simulink model "LoadFlow116BusNetwork_original"  (R2024a)
settings: Solver=FixedStepDiscrete  StartTime=0.0  StopTime=4.5  FixedStep=75e-6  RelTol=1e-3  EnableMultiTasking=on
undefined symbols (not defined in the file or in its folder): D1, D11, Delta
libraries: spsSeriesRLCBranchLib x164, spsLoadFlowBusLib x116, spsDistributedParametersLineLib x79, spsThreePhaseSeriesRLCLoadLib x60, spsThreePhaseTransformerTwoWindingsLib x52, spsThreePhaseParallelRLCLoadLib x44, spsThreePhaseVIMeasurementLib x44, spsSynchronousMachinepuStandardLib x28, spsExcitationSystemLib x28, spsHydraulicTurbineandGovernorLib x28, spsGenericPowerSystemStabilizerLib x28, spsMultiBandPowerSystemStabilizerLib x28
(part 3 of 15)

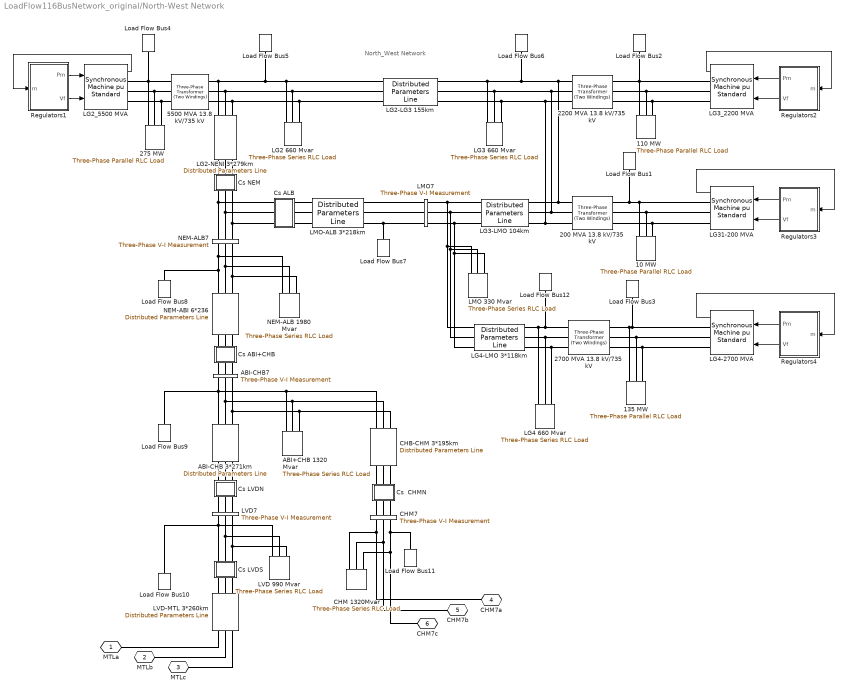
== system LoadFlow116BusNetwork_original/North-West Network ==
  note: North_West Network
  10 MW : spsThreePhaseParallelRLCLoadLib/Three-Phase Parallel RLC Load  LConnTagsString=A|B|C  Configuration=Y (grounded)  NominalVoltage=(13800)*1  Vabc=[1e3 1e3 1e3]  Vabcp=[1e3 1e3 1e3]  NominalFrequency=60  UnbalancedPower=off  ActivePower=10000000  InductivePower=0  CapacitivePower=0  Pabc=[10e3 9e3 11e3]  QLabc=[100 90 110]  QCabc=[100 90 110]  Pabcp=[10e3 9e3 11e3]  QLabcp=[100 90 110]  QCabcp=[100 90 110]  Measurements=None  LoadType=constant PQ
  110 MW : spsThreePhaseParallelRLCLoadLib/Three-Phase Parallel RLC Load  LConnTagsString=A|B|C  Configuration=Y (grounded)  NominalVoltage=(13800)*1  Vabc=[1e3 1e3 1e3]  Vabcp=[1e3 1e3 1e3]  NominalFrequency=60  UnbalancedPower=off  ActivePower=110000000  InductivePower=0  CapacitivePower=0  Pabc=[10e3 9e3 11e3]  QLabc=[100 90 110]  QCabc=[100 90 110]  Pabcp=[10e3 9e3 11e3]  QLabcp=[100 90 110]  QCabcp=[100 90 110]  Measurements=None  LoadType=constant PQ
  135 MW : spsThreePhaseParallelRLCLoadLib/Three-Phase Parallel RLC Load  LConnTagsString=A|B|C  Configuration=Y (grounded)  NominalVoltage=(13800)*1  Vabc=[1e3 1e3 1e3]  Vabcp=[1e3 1e3 1e3]  NominalFrequency=60  UnbalancedPower=off  ActivePower=135000000  InductivePower=0  CapacitivePower=0  Pabc=[10e3 9e3 11e3]  QLabc=[100 90 110]  QCabc=[100 90 110]  Pabcp=[10e3 9e3 11e3]  QLabcp=[100 90 110]  QCabcp=[100 90 110]  Measurements=None  LoadType=constant PQ
  200 MVA 13.8 kV/735 kV : spsThreePhaseTransformerTwoWindingsLib/Three-Phase Transformer (Two Windings)  Winding1Connection=Delta (D1)  Winding2Connection=Yg  CoreType=Three single-phase transformers  SetSaturation=off  Hysteresis=off  DataFile='basic_model'  SetInitialFlux=off  Measurements=None  UNITS=pu  NominalPower=[ 200e6 60 ]  Winding1="[ 13.8e3 0.002  0.0]"  Winding2=[ 735e3 0.002 0.12]  Rm=500  Lm=500  L0=0.5  Saturation="[ 0,0  ;  0.005,1.2  ;  1.0,1.4 ]"  InitialFluxes=[ 0.8 , -0.8 , 0.7 ]  BreakLoop=off  DiscreteSolver=Trapezoidal iterative  DataType=off  TransfoNumber=0
  2200 MVA 13.8 kV/735 kV : spsThreePhaseTransformerTwoWindingsLib/Three-Phase Transformer (Two Windings)  Winding1Connection=Delta (D1)  Winding2Connection=Yg  CoreType=Three single-phase transformers  SetSaturation=off  Hysteresis=off  DataFile='basic_model'  SetInitialFlux=off  Measurements=None  UNITS=pu  NominalPower=[ 2200e6 60 ]  Winding1="[ 13.8e3 0.002  0.0]"  Winding2=[ 735e3 0.002 0.12]  Rm=500  Lm=500  L0=0.5  Saturation="[ 0,0  ;  0.005,1.2  ;  1.0,1.4 ]"  InitialFluxes=[ 0.8 , -0.8 , 0.7 ]  BreakLoop=off  DiscreteSolver=Trapezoidal iterative  DataType=off  TransfoNumber=0
  2700 MVA 13.8 kV/735 kV : spsThreePhaseTransformerTwoWindingsLib/Three-Phase Transformer (Two Windings)  Winding1Connection=Delta (D1)  Winding2Connection=Yg  CoreType=Three single-phase transformers  SetSaturation=off  Hysteresis=off  DataFile='basic_model'  SetInitialFlux=off  Measurements=None  UNITS=pu  NominalPower=[ 2700e6 60 ]  Winding1="[ 13.8e3 0.002  0.0]"  Winding2=[ 735e3 0.002 0.12]  Rm=500  Lm=500  L0=0.5  Saturation="[ 0,0  ;  0.005,1.2  ;  1.0,1.4 ]"  InitialFluxes=[ 0.8 , -0.8 , 0.7 ]  BreakLoop=off  DiscreteSolver=Trapezoidal iterative  DataType=off  TransfoNumber=0
  275 MW : spsThreePhaseParallelRLCLoadLib/Three-Phase Parallel RLC Load  LConnTagsString=A|B|C  Configuration=Y (grounded)  NominalVoltage=(13800)*1  Vabc=[1e3 1e3 1e3]  Vabcp=[1e3 1e3 1e3]  NominalFrequency=60  UnbalancedPower=off  ActivePower=275000000  InductivePower=0  CapacitivePower=0  Pabc=[10e3 9e3 11e3]  QLabc=[100 90 110]  QCabc=[100 90 110]  Pabcp=[10e3 9e3 11e3]  QLabcp=[100 90 110]  QCabcp=[100 90 110]  Measurements=None  LoadType=constant PQ
  5500 MVA 13.8 kV/735 kV : spsThreePhaseTransformerTwoWindingsLib/Three-Phase Transformer (Two Windings)  Winding1Connection=Delta (D1)  Winding2Connection=Yg  CoreType=Three single-phase transformers  SetSaturation=off  Hysteresis=off  DataFile='basic_model'  SetInitialFlux=off  Measurements=None  UNITS=pu  NominalPower=[ 5500e6 60 ]  Winding1="[ 13.8e3 0.002  0.0]"  Winding2=[ 735e3 0.002 0.12]  Rm=500  Lm=500  L0=0.5  Saturation="[ 0,0  ;  0.005,1.2  ;  1.0,1.4 ]"  InitialFluxes=[ 0.8 , -0.8 , 0.7 ]  BreakLoop=off  DiscreteSolver=Trapezoidal iterative  DataType=off  TransfoNumber=0
  ABI+CHB 1320 Mvar : spsThreePhaseSeriesRLCLoadLib/Three-Phase Series RLC Load  LConnTagsString=A|B|C  Configuration=Y (grounded)  NominalVoltage=735e3  Vabc=[1e3 1e3 1e3]  Vabcp=[1e3 1e3 1e3]  NominalFrequency=60  UnbalancedPower=off  ActivePower=4400000  InductivePower=1320e6  CapacitivePower=0  Pabc=[10e3 9e3 11e3]  QLabc=[100 90 110]  QCabc=[100 90 110]  Pabcp=[10e3 9e3 11e3]  QLabcp=[100 90 110]  QCabcp=[100 90 110]  Measurements=None  LoadType=constant Z
  ABI-CHB 3*271km : spsDistributedParametersLineLib/Distributed Parameters Line  Phases=3  Length=271  Frequency=60  Resistance="[0.01273  0.3864]/3"  Inductance="[0.9337e-3  4.1264e-3]/3"  Capacitance=[12.74e-9 7.751e-9]*3  x1=[-0.001575 3.83249072532594e-08 -6095.79039966501 -646119.037388301;-0.0015 3.82765773827991e-08 12172.7797950193 -646033.103735147;-0.001425 3.81976498020301e-08 30431.6192557852 -645430.741103505;-0.00135 3.80881876044531e-08 48666.1321457375 -644312.431012847;-0.001275 3.79482782924739e-08 66861.7420742692 -642679.067423147;-0.0012 3.77780337074559e-08 85003.9037492058 -640531.956020269;-0.001125 3.75775899403154e-08 103078.114604089 -637872.813172216;-0.00105 3.7347107222733e-08 121069.926391305 -634703.764557095;-0.000975 3.70867697990666e-08 138964.956731796 -631027.343463879;-0.0009 3.67967857790695e-08 156748.900612111 -626846.488767341;-0.000825 3.64773869715303e-08 174407.541819615 -622164.542578755;-0.00075 3.61288286989688e-08 191926.764306713 -616985.247574268;-0.000675 3.5751389593535e-08 209292.563475003 -611312.744003061;-0.0006 3.53453713742747e-08 226491.057370334 -605151.566377697;-0.000525 3.49110986059401e-08 243508.497779833 -598506.6398493;-0.00045 3.44489184395376e-08 260331.281222011 -591383.276270467;-0.000375 3.39592003348207e-08 276945.959821183 -583787.16994905;-0.0003 3.34423357649494e-08 293339.252057489 -575724.393096219;-0.000225 3.28987379035524e-08 309498.053383942 -567201.390972425;-0.00015 3.23288412944429e-08 325409.446701998 -558224.976735161;-7.5e-05 3.17331015042505e-08 341060.712687292 -548802.325992623]  x2=[-0.001575 8.2065527540125e-08 -248614.692980884 -602078.188381389;-0.0015 8.19104771840523e-08 -231494.235349716 -608866.016701668;-0.001425 8.1689948845791e-08 -214188.724768791 -615167.126844157;-0.00135 8.14041188123205e-08 -196711.994998483 -620976.48179782;-0.001275 8.10532155717962e-08 -179078.016669168 -626289.437653192;-0.0012 8.06375196308996e-08 -161300.886113313 -631101.747314655;-0.001125 8.01573632906055e-08 -143394.814097085 -635409.563895494;-0.00105 7.96131303805457e-08 -125374.114460482 -639209.443793048;-0.000975 7.90052559521814e-08 -107253.192675068 -642498.349441466;-0.0009 7.83342259310298e-08 -89046.5343284583 -645273.651739895;-0.000825 7.76005767282229e-08 -70768.6935447641 -647533.132154141;-0.00075 7.6804894811708e-08 -52434.2813502475 -649274.984490132;-0.000675 7.5947816237435e-08 -34057.9539934908 -650497.816337762;-0.0006 7.50300261409023e-08 -15654.401229416 -651200.650183962;-0.000525 7.40522581894705e-08 2761.66542348126 -651382.924194109;-0.00045 7.30152939958796e-08 21175.5244432939 -651044.492661148;-0.000375 7.19199624934398e-08 39572.4560728629 -650185.626122069;-0.0003 7.07671392733951e-08 57937.7540865262 -648807.011141641;-0.000225 6.95577458849888e-08 76256.7375460501 -646909.749763587;-0.00015 6.82927490987912e-08 94514.7625363469 -644495.358629623;-7.5e-05 6.69731601338781e-08 112697.233871596 -641565.767767081]  x3=[-0.001575 2.28122692087179e-10 -202.312158706382 698.106439471975;-0.0015 2.37186669278141e-10 -221.966976543685 692.108516416584;-0.001425 2.4606104307476e-10 -241.444357376149 685.557332402785;-0.00135 2.54738719438405e-10 -260.728731283548 678.458124346841;-0.001275 2.63212761567364e-10 -279.804682632443 670.816567247053;-0.0012 2.71476395442016e-10 -298.656962399196 662.638769647245;-0.001125 2.7952301523988e-10 -317.270500359813 653.931268753694;-0.00105 2.87346188616207e-10 -335.630417136843 644.701025209385;-0.000975 2.94939661845898e-10 -353.722036093731 634.95541752978;-0.0009 3.02297364822638e-10 -371.530895067095 624.702236204546;-0.000825 3.09413415911243e-10 -389.042757927556 613.949677469955;-0.00075 3.16282126649353e-10 -406.243625959883 602.706336756939;-0.000675 3.22898006294698e-10 -423.119749053353 590.981201820035;-0.0006 3.29255766214317e-10 -439.65763669338 578.783645552713;-0.000525 3.35350324112206e-10 -455.844068745621 566.123418494822;-0.00045 3.41176808092031e-10 -471.666106023956 553.010641038166;-0.000375 3.46730560551648e-10 -487.111100633868 539.455795336409;-0.0003 3.52007141906316e-10 -502.166706082983 525.469716925812;-0.000225 3.57002334137633e-10 -516.820887150664 511.06358606346;-0.00015 3.6171214416536e-10 -531.061929508781 496.248918789945;-7.5e-05 3.66132807039422e-10 -544.878449085969 481.037557723611]  x4=[-0.001575 2.1639318364885e-10 -5039.99478840233 -13897.9312159908;-0.0015 2.10323530529909e-10 -4645.07840312812 -14034.8602322776;-0.001425 2.04085747998721e-10 -4246.44881325052 -14160.5699960354;-0.00135 1.97684822443198e-10 -3844.42467716446 -14274.9600168023;-0.001275 1.91125870665294e-10 -3439.32736681315 -14377.938852946;-0.0012 1.84414135790704e-10 -3031.48071078828 -14469.4241847605;-0.001125 1.77554983077594e-10 -2621.21073546641 -14549.3428802713;-0.00105 1.70553895627694e-10 -2208.84540438848 -14617.631053696;-0.000975 1.63416470003191e-10 -1794.71435609076 -14674.2341165137;-0.0009 1.56148411752923e-10 -1379.14864059682 -14719.1068211019;-0.000825 1.48755530851451e-10 -962.480454781271 -14752.2132969072;-0.00075 1.41243737054653e-10 -545.042876816616 -14773.5270791194;-0.000675 1.33619035175554e-10 -127.169599915668 -14783.0311298271;-0.0006 1.25887520284176e-10 290.805334417691 -14780.7178516376;-0.000525 1.18055372835226e-10 708.547803416187 -14766.5890937501;-0.00045 1.1012885372754e-10 1125.72387014178 -14740.6561504774;-0.000375 1.02114299299212e-10 1542.00005042973 -14702.9397522176;-0.0003 9.40181162624252e-11 1957.04357947076 -14653.4700488824;-0.000225 8.58467765820237e-11 2370.52267781813 -14592.2865857957;-0.00015 7.76068123019223e-11 2782.10681660707 -14519.4382720818;-7.5e-05 6.93048103234907e-11 3191.46698177448 -14434.9833415681]  x5=0.00153261764655846  V1=ones(3,3)  V2=ones(3,3)  I1=ones(3,3)  I2=ones(3,3)  nHarmo=1  Measurements=None  Decoupling=off  VsMag0=[ 1 1 1]  VrMag0=[ 1 1 1]  VsAngle0=[0 -120 120]  VrAngle0=[0 -120 120]  IsMag0=[ 1 1 1]  IrMag0=[ 1 1 1]  IsAngle0=[0 -120 120]  IrAngle0=[0 -120 120]
      settings: AttributesFormatString=\n  LibrarySourceBlock=sps_lib/Power Grid Elements/Distributed Parameters Line
  ABI-CHB7 : spsThreePhaseVIMeasurementLib/Three-Phase V-I Measurement  VoltageMeasurement=no  SetLabelV=on  LabelV=Vabc_ABI7  Vpu=on  VpuLL=off  CurrentMeasurement=no  SetLabelI=off  LabelI=A1  Ipu=off  Pbase=100e6  Vbase=500e3  OutputType=Magnitude  PhasorSimulation=off  PSBequivalent=0
  CHB-CHM 3*195km : spsDistributedParametersLineLib/Distributed Parameters Line  Phases=3  Length=195  Frequency=60  Resistance="[0.01273  0.3864]/3"  Inductance="[0.9337e-3  4.1264e-3]/3"  Capacitance=[12.74e-9 7.751e-9]*3  x1=[-0.001125 3.75775899403154e-08 0 0;-0.00105 3.7347107222733e-08 0 0;-0.000975 3.70867697990666e-08 0 0;-0.0009 3.67967857790695e-08 0 0;-0.000825 3.64773869715303e-08 0 0;-0.00075 3.61288286989688e-08 0 0;-0.000675 3.5751389593535e-08 209292.563475003 -611312.744003061;-0.0006 3.53453713742747e-08 226491.057370334 -605151.566377697;-0.000525 3.49110986059401e-08 243508.497779833 -598506.6398493;-0.00045 3.44489184395376e-08 260331.281222011 -591383.276270467;-0.000375 3.39592003348207e-08 276945.959821183 -583787.16994905;-0.0003 3.34423357649494e-08 293339.252057489 -575724.393096219;-0.000225 3.28987379035524e-08 309498.053383942 -567201.390972425;-0.00015 3.23288412944429e-08 325409.446701998 -558224.976735161;-7.5e-05 3.17331015042505e-08 341060.712687292 -548802.325992623]  x2=[-0.001125 2.54585987102807e-08 0 0;-0.00105 2.52619775854315e-08 0 0;-0.000975 2.50451624222217e-08 0 0;-0.0009 2.48083265393754e-08 0 0;-0.000825 2.45516592598736e-08 0 0;-0.00075 2.42753657596125e-08 0 0;-0.000675 2.39796669033887e-08 111004.534524873 -639558.940614557;-0.0006 2.36647990683436e-08 129040.856793954 -636165.151877404;-0.000525 2.33310139550067e-08 146974.025776505 -632262.822451493;-0.00045 2.29785783860908e-08 164789.705971629 -627855.071799261;-0.000375 2.2607774093197e-08 182473.655797166 -622945.423409136;-0.0003 2.22188974916037e-08 200011.738974199 -617537.801978923;-0.000225 2.18122594433161e-08 217389.935827378 -611636.530278454;-0.00015 2.13881850085683e-08 234594.354492034 -605246.325694032;-7.5e-05 2.09470131859748e-08 251611.242019124 -598372.29645743]  x3=[-0.001125 1.1406073283713e-10 0 0;-0.00105 1.11027071751763e-10 0 0;-0.000975 1.0790465732401e-10 0 0;-0.0009 1.04695985564188e-10 0 0;-0.000825 1.01403621435409e-10 0 0;-0.00075 9.80301968031813e-11 0 0;-0.000675 9.45784083315417e-11 49.2476883451521 -2749.35029594692;-0.0006 9.105101532738e-11 126.954449514307 -2746.85863034019;-0.000525 8.74508375346929e-11 204.559725238988 -2742.17116797272;-0.00045 8.37807528805233e-11 282.001479049181 -2735.29165593019;-0.000375 8.00436951743894e-11 359.21780519179 -2726.22559358927;-0.0003 7.62426517630428e-11 436.146978117146 -2714.98022822149;-0.000225 7.23806611424285e-11 512.727501821467 -2701.56454919986;-0.00015 6.84608105287581e-11 588.898159005826 -2685.98928081293;-7.5e-05 6.44862333906367e-11 664.59806001232 -2668.26687369192]  x4=[-0.001125 1.40123928232881e-10 0 0;-0.00105 1.43102353076615e-10 0 0;-0.000975 1.45966384088839e-10 0 0;-0.0009 1.48713731806983e-10 0 0;-0.000825 1.51342200043317e-10 0 0;-0.00075 1.53849687640549e-10 0 0;-0.000675 1.56234190151461e-10 1717.04187839558 -11467.1483442359;-0.0006 1.58493801441229e-10 2040.53742261583 -11414.0235556932;-0.000525 1.60626715211161e-10 2362.40179244172 -11351.7745713605;-0.00045 1.62631226442625e-10 2682.37769442068 -11280.4511521235;-0.000375 1.64505732760011e-10 3000.20934471248 -11200.1103128321;-0.0003 1.66248735711652e-10 3315.64267355886 -11110.8162767241;-0.000225 1.67858841967655e-10 3628.42552838303 -11012.6404240857;-0.00015 1.69334764433716e-10 3938.30787535659 -10905.6612351913;-7.5e-05 1.70675323279997e-10 4245.04199927271 -10789.9642275676]  x5=0.0011028060556417  V1=ones(3,3)  V2=ones(3,3)  I1=ones(3,3)  I2=ones(3,3)  nHarmo=1  Measurements=None  Decoupling=off  VsMag0=[ 1 1 1]  VrMag0=[ 1 1 1]  VsAngle0=[0 -120 120]  VrAngle0=[0 -120 120]  IsMag0=[ 1 1 1]  IrMag0=[ 1 1 1]  IsAngle0=[0 -120 120]  IrAngle0=[0 -120 120]
      settings: AttributesFormatString=\n  LibrarySourceBlock=sps_lib/Power Grid Elements/Distributed Parameters Line
  CHM 1320Mvar : spsThreePhaseSeriesRLCLoadLib/Three-Phase Series RLC Load  LConnTagsString=A|B|C  Configuration=Y (grounded)  NominalVoltage=735e3  Vabc=[1e3 1e3 1e3]  Vabcp=[1e3 1e3 1e3]  NominalFrequency=60  UnbalancedPower=off  ActivePower=4400000  InductivePower=1320e6  CapacitivePower=0  Pabc=[10e3 9e3 11e3]  QLabc=[100 90 110]  QCabc=[100 90 110]  Pabcp=[10e3 9e3 11e3]  QLabcp=[100 90 110]  QCabcp=[100 90 110]  Measurements=None  LoadType=constant Z
  CHM7 : spsThreePhaseVIMeasurementLib/Three-Phase V-I Measurement  VoltageMeasurement=no  SetLabelV=on  LabelV=Vabc_CHM7  Vpu=on  VpuLL=off  CurrentMeasurement=no  SetLabelI=off  LabelI=A1  Ipu=off  Pbase=100e6  Vbase=735e3  OutputType=Magnitude  PhasorSimulation=off  PSBequivalent=0
  "Cs  CHMN " : Subsystem  mask{Xc=25/3}
      mask prompts: Xc "Condensator Reactance at  60Hz  (ohm):"
      mask help: Series Compensation
      mask init:
      | Cs=1/Xc/(2*pi*60);
      mask Display: disp('Cs')
  "Cs ABI+CHB " : Subsystem  mask{Xc=25/6}
      mask prompts: Xc "Condensator Reactance at  60Hz  (ohm):"
      mask help: Series Compensation
      mask init:
      | Cs=1/Xc/(2*pi*60);
      mask Display: disp('Cs')
  Cs ALB : Subsystem  mask{Xc=16/3}
      mask prompts: Xc "Reactance @ 60Hz du condensateur (ohm):"
      mask init:
      | Cs=1/Xc/(2*pi*60);
      mask Display: disp('Cs')
  "Cs LVDN " : Subsystem  mask{Xc=34/3}
      mask prompts: Xc "Condensator Reactance at  60Hz  (ohm):"
      mask help: Series Compensation
      mask init:
      | Cs=1/Xc/(2*pi*60);
      mask Display: disp('Cs')
  "Cs LVDS " : Subsystem  mask{Xc=34/3}
      mask prompts: Xc "Condensator Reactance at  60Hz  (ohm):"
      mask help: Series Compensation
      mask init:
      | Cs=1/Xc/(2*pi*60);
      mask Display: disp('Cs')
  "Cs NEM " : Subsystem  mask{Xc=16/3}
      mask prompts: Xc "Condensator Reactance at  60Hz  (ohm):"
      mask help: Series Compensation
      mask init:
      | Cs=1/Xc/(2*pi*60);
      mask Display: disp('Cs')
  LG2 660 Mvar : spsThreePhaseSeriesRLCLoadLib/Three-Phase Series RLC Load  LConnTagsString=A|B|C  Configuration=Y (grounded)  NominalVoltage=735e3  Vabc=[1e3 1e3 1e3]  Vabcp=[1e3 1e3 1e3]  NominalFrequency=60  UnbalancedPower=off  ActivePower=2200000  InductivePower=660e6  CapacitivePower=0  Pabc=[10e3 9e3 11e3]  QLabc=[100 90 110]  QCabc=[100 90 110]  Pabcp=[10e3 9e3 11e3]  QLabcp=[100 90 110]  QCabcp=[100 90 110]  Measurements=None  LoadType=constant Z
  LG2-LG3 155km : spsDistributedParametersLineLib/Distributed Parameters Line  Phases=3  Length=155  Frequency=60  Resistance="[0.01273  0.3864]"  Inductance="[0.9337e-3  4.1264e-3]"  Capacitance=[12.74e-9 7.751e-9]  x1=[-0.0009 -4.84332126491647e-12 431553.276717606 -473538.091690277;-0.000825 -1.18699024701789e-11 444767.94531887 -461148.506915093;-0.00075 -1.88869950570223e-11 457627.073229824 -448390.287079289;-0.000675 -2.58889896689978e-11 470120.381060367 -435273.630908595;-0.0006 -3.28702890187468e-11 482237.881851374 -421809.023657264;-0.000525 -3.98253123623864e-11 493969.889058115 -408007.228726315;-0.00045 -4.67484999606713e-11 505307.024293536 -393879.279059442;-0.000375 -5.36343175233636e-11 516240.224825194 -379436.468323444;-0.0003 -6.04772606332604e-11 526760.750819866 -364690.34188024;-0.000225 -6.727185914634e-11 536860.192330043 -349652.687557688;-0.00015 -7.4012681564512e-11 546530.476016708 -334335.526226567;-7.5e-05 -8.06943393774733e-11 555763.871603042 -318751.102191285]  x2=[-0.0009 -3.13192936908636e-10 434484.753049099 -467489.581126943;-0.000825 -3.72034271017443e-10 447527.255752058 -455019.542461733;-0.00075 -4.30578206622315e-10 460212.012014165 -442185.768136312;-0.000675 -4.88777944596881e-10 472528.881835348 -428998.517273512;-0.0006 -5.46586960961089e-10 484468.019298325 -415468.331559901;-0.000525 -6.03959044071765e-10 496019.880439286 -401606.026818919;-0.00045 -6.60848331563494e-10 507175.230877181 -387422.684364877;-0.000375 -7.17209347010289e-10 517925.153195555 -372929.642144719;-0.0003 -7.72997036278756e-10 528261.054070985 -358138.485674646;-0.000225 -8.28166803543673e-10 538174.671142455 -343061.038778827;-0.00015 -8.82674546937213e-10 547658.079616163 -327709.354137618;-7.5e-05 -9.36476693803306e-10 556703.698600475 -312095.703652833]  x3=[-0.0009 6.67600828525714e-12 1522.16056329695 -1950.05893522514;-0.000825 6.53713605124591e-12 1576.68135164252 -1906.24695426415;-0.00075 6.39303813069686e-12 1629.94176503962 -1860.91114865447;-0.000675 6.24382971328289e-12 1681.89922792869 -1814.08775914546;-0.0006 6.08963007392992e-12 1732.51220630888 -1765.81421563826;-0.000525 5.93056247747032e-12 1781.74024093967 -1716.12910726494;-0.00045 5.76675408010688e-12 1829.5439796834 -1665.07215154092;-0.000375 5.59833582776609e-12 1875.88520896272 -1612.68416261543;-0.0003 5.425442351422e-12 1920.72688430801 -1559.00701864523;-0.000225 5.24821185947424e-12 1964.03315997009 -1504.08362831794;-0.00015 5.06678602726634e-12 2005.7694175748 -1447.95789655142;-7.5e-05 4.88130988383267e-12 2045.90229379641 -1390.6746893969]  x4=[-0.0009 -8.09837001596585e-12 1309.19110331862 -1829.24101140865;-0.000825 -8.05817320331329e-12 1360.38131280614 -1791.49811725832;-0.00075 -8.01153481029618e-12 1410.48405428674 -1752.3231269239;-0.000675 -7.95849211893232e-12 1459.45927639548 -1711.74735629325;-0.0006 -7.8990875307376e-12 1507.26782908914 -1669.8032410166;-0.000525 -7.83336853283089e-12 1553.8714949422 -1626.52431057793;-0.00045 -7.7613876599736e-12 1599.23301969723 -1581.94516149203;-0.000375 -7.68320245257414e-12 1643.3161420454 -1536.10142964861;-0.0003 -7.59887541069103e-12 1686.0856226132 -1489.02976182547;-0.000225 -7.5084739440713e-12 1727.50727213226 -1440.76778639365;-0.00015 -7.41207031826419e-12 1767.54797876972 -1391.35408323787;-7.5e-05 -7.30974159685314e-12 1806.17573459735 -1340.82815291638]  x5=0.000876589428843401  V1=ones(3,3)  V2=ones(3,3)  I1=ones(3,3)  I2=ones(3,3)  nHarmo=1  Measurements=None  Decoupling=off  VsMag0=[ 1 1 1]  VrMag0=[ 1 1 1]  VsAngle0=[0 -120 120]  VrAngle0=[0 -120 120]  IsMag0=[ 1 1 1]  IrMag0=[ 1 1 1]  IsAngle0=[0 -120 120]  IrAngle0=[0 -120 120]
      settings: AttributesFormatString=\n  LibrarySourceBlock=sps_lib/Power Grid Elements/Distributed Parameters Line
  LG2-NENI 3*279km : spsDistributedParametersLineLib/Distributed Parameters Line  Phases=3  Length=279  Frequency=60  Resistance="[0.01273  0.3864]/3"  Inductance="[0.9337e-3  4.1264e-3]/3"  Capacitance=[12.74e-9 7.751e-9]*3  x1=[-0.00165 6.47106599077037e-11 282305.297313516 -575135.752528798;-0.001575 5.78971545940454e-11 298451.827359396 -566924.896508542;-0.0015 5.10373671808608e-11 314359.779580952 -558260.849400258;-0.001425 4.41367812772497e-11 330016.437404577 -549150.537110641;-0.00135 3.7200913106001e-11 345409.285137561 -539601.242283943;-0.001275 3.02353070940084e-11 360526.017972946 -529620.598480339;-0.0012 2.32455314401406e-11 375354.551825796 -519216.584073777;-0.001125 1.62371736641081e-11 389883.032993033 -508397.515874186;-0.00105 9.21583613988556e-12 404099.847629107 -497172.042479149;-0.000975 2.18713161725983e-12 417993.631029921 -485549.13736034;-0.0009 -4.84332126491649e-12 431553.276717606 -473538.091690277;-0.000825 -1.18699024701789e-11 444767.94531887 -461148.506915093;-0.00075 -1.88869950570223e-11 457627.073229824 -448390.287079289;-0.000675 -2.58889896689978e-11 470120.381060367 -435273.630908595;-0.0006 -3.28702890187468e-11 482237.881851374 -421809.023657264;-0.000525 -3.98253123623864e-11 493969.889058115 -408007.228726314;-0.00045 -4.67484999606713e-11 505307.024293536 -393879.279059442;-0.000375 -5.36343175233636e-11 516240.224825194 -379436.468323444;-0.0003 -6.04772606332604e-11 526760.750819866 -364690.34188024;-0.000225 -6.727185914634e-11 536860.192330043 -349652.687557688;-0.00015 -7.4012681564512e-11 546530.476016708 -334335.526226567;-7.5e-05 -8.06943393774733e-11 555763.871603042 -318751.102191285]  x2=[-0.00165 2.24543208818106e-08 59028.0607461738 -635612.64855906;-0.001575 2.24509751096562e-08 76973.5739081375 -633689.821780446;-0.0015 2.24296823715106e-08 94857.5555728542 -631260.433054081;-0.001425 2.23904596884629e-08 112665.709559015 -628326.42439614;-0.00135 2.23333384145257e-08 130383.800300798 -624890.141208254;-0.001275 2.22583642115715e-08 147997.664227559 -620954.330402626;-0.0012 2.2165597012831e-08 165493.221085977 -616522.138206193;-0.001125 2.20551109749834e-08 182856.48519559 -611597.107645584;-0.00105 2.19269944188769e-08 200073.576628736 -606183.175714872;-0.000975 2.17813497589262e-08 217130.732305953 -600284.670228408;-0.0009 2.16182934212441e-08 234014.316997976 -593906.306361226;-0.000825 2.1437955750572e-08 250710.834225531 -587053.182879811;-0.00075 2.12404809060847e-08 267206.937048209 -579730.778066216;-0.000675 2.10260267461512e-08 283489.438733815 -571944.945338813;-0.0006 2.07947647021459e-08 299545.323299631 -563701.908573158;-0.000525 2.05468796414083e-08 315361.755917198 -555008.257126718;-0.00045 2.02825697194631e-08 330926.093172281 -545870.940571442;-0.000375 2.00020462216179e-08 346225.893171822 -536297.263138378;-0.0003 1.97055333940647e-08 361248.925489795 -526294.877878785;-0.000225 1.93932682646211e-08 375983.180944025 -515871.780546397;-0.00015 1.90655004532537e-08 390416.881196144 -505036.303205743;-7.5e-05 1.87224919725359e-08 404538.488167014 -493797.107571622]  x3=[-0.00165 3.07334969874037e-11 -180.946605754108 -28.0430826418668;-0.001575 3.47618796909601e-11 -180.081241438496 -33.1461710862671;-0.0015 3.87624742797662e-11 -179.071922933813 -38.2227629886544;-0.001425 4.27320827397188e-11 -177.91945707383 -43.2688001991364;-0.00135 4.66675318265521e-11 -176.62476512212 -48.2802489927741;-0.001275 5.05656756024803e-11 -175.188882035622 -53.2531032940795;-0.0012 5.44233979510128e-11 -173.612955637304 -58.1833878794115;-0.001125 5.82376150679291e-11 -171.898245698617 -63.0671615547084;-0.00105 6.20052779264255e-11 -170.046122932449 -67.9005203060183;-0.000975 6.57233747144601e-11 -168.058067897403 -72.6796004203084;-0.0009 6.93889332423493e-11 -165.935669814254 -77.4005815740577;-0.000825 7.29990233186908e-11 -163.680625295556 -82.0596898871653;-0.00075 7.65507590927139e-11 -161.294736989394 -86.6532009397325;-0.000675 8.00413013611842e-11 -158.779912138376 -91.1774427493069;-0.0006 8.34678598380193e-11 -156.138161055008 -95.6287987062091;-0.000525 8.6827695384801e-11 -153.371595514687 -100.003710464595;-0.00045 9.01181222004003e-11 -150.482427067575 -104.298680786944;-0.000375 9.33365099679662e-11 -147.472965270724 -108.510276339695;-0.0003 9.64802859575602e-11 -144.345615841848 -112.635130437803;-0.000225 9.95469370827576e-11 -141.102878736229 -116.669945736015;-0.00015 1.0253401190957e-10 -137.747346148296 -120.611496864715;-7.5e-05 1.05439122616085e-10 -134.281700439456 -124.456633008239]  x4=[-0.00165 5.23544330679684e-11 1481.48089108623 -13945.3845775462;-0.001575 4.89577475050573e-11 1875.13150496137 -13897.9289700668;-0.0015 4.55219258678693e-11 2267.28316740192 -13839.3635708141;-0.001425 4.20497146996513e-11 2657.62239836904 -13769.7351960722;-0.00135 3.85438896328847e-11 3045.8371666539 -13689.0995056986;-0.001275 3.50072531704868e-11 3431.6171393106 -13597.5209586304;-0.0012 3.14426324455333e-11 3814.65392973164 -13495.0727613569;-0.001125 2.78528769612913e-11 4194.64134416741 -13381.8368093996;-0.00105 2.42408563133698e-11 4571.27562649282 -13257.9036218457;-0.000975 2.06094578958089e-11 4944.25570102528 -13123.3722689893;-0.0009 1.69615845929414e-11 5313.28341319998 -12978.3502931354;-0.000825 1.33001524588712e-11 5678.06376791014 -12822.9536226326;-0.00075 9.62808838642453e-12 6038.30516532152 -12657.3064792016;-0.000675 5.94832776743645e-12 6393.7196339729 -12481.5412786344;-0.0006 2.26381214624357e-12 6744.02306097608 -12295.7985249431;-0.000525 -1.42251313174154e-12 7088.93541913133 -12100.226698043;-0.00045 -5.10770127449432e-12 7428.18099077687 -11894.9821350601;-0.000375 -8.78880639899871e-12 7761.48858819337 -11680.2289053577;-0.0003 -1.2462885886141e-11 8088.59177038722 -11456.138679382;-0.000225 -1.61270027329944e-11 8409.22905607943 -11222.8905914307;-0.00015 -1.97782279006146e-11 8723.14413272973 -10980.6710964566;-7.5e-05 -2.3413642655468e-11 9030.08606142891 -10729.673821018]  x5=0.00157786097191812  V1=ones(3,3)  V2=ones(3,3)  I1=ones(3,3)  I2=ones(3,3)  nHarmo=1  Measurements=None  Decoupling=off  VsMag0=[ 1 1 1]  VrMag0=[ 1 1 1]  VsAngle0=[0 -120 120]  VrAngle0=[0 -120 120]  IsMag0=[ 1 1 1]  IrMag0=[ 1 1 1]  IsAngle0=[0 -120 120]  IrAngle0=[0 -120 120]
      settings: AttributesFormatString=\n  LibrarySourceBlock=sps_lib/Power Grid Elements/Distributed Parameters Line
  LG2_5500 MVA : spsSynchronousMachinepuStandardLib/Synchronous Machine pu Standard  PresetModel=No  MechanicalLoad=Mechanical power Pm  ShowDetailedParameters=on  RotorType=Salient-pole  Units=per unit standard parameters  MeasurementBus=off  NominalParameters="[5500E6  13800   60 ]"  Reactances1=[ 31 32 33 34 35 36 37 ]  Reactances2=[ 1.305, 0.296, 0.252, 0.474, 0.243, 0.18 ]  dAxisTimeConstants=Short-circuit  qAxisTimeConstants=Open-circuit  TimeConstants1=[]  TimeConstants2=[]  TimeConstants3=[]  TimeConstants4=[]  TimeConstants5=[ 1.01, 0.053, 0.1 ]  TimeConstants6=[]  TimeConstants7=[]  TimeConstants8=[]  StatorResistance=2.8544e-3  Mechanical="[ 4.1  0  32]"  PolePairs=32  InitialConditions=[0 -65.2434 0.985682 0.985682 0.985682 -1.22427 -121.224 118.776 1.47412]  SetSaturation=off  Saturation=[0.6404,0.7127,0.8441,0.9214,0.9956,1.082,1.19,1.316,1.457;0.7,0.7698,0.8872,0.9466,0.9969,1.046,1.1,1.151,1.201]  LoadFlowParameters=[2 4000000000 0 0 0]  TsPowergui=0  TsBlock=-1  IterativeModel=Trapezoidal non iterative  IterativeDiscreteModel=Trapezoidal non iterative  BusType=swing  Pref=0  Qref=0  Qmin=-Inf  Qmax=Inf  PLF=0  QLF=0
  LG3 660 Mvar : spsThreePhaseSeriesRLCLoadLib/Three-Phase Series RLC Load  LConnTagsString=A|B|C  Configuration=Y (grounded)  NominalVoltage=735e3  Vabc=[1e3 1e3 1e3]  Vabcp=[1e3 1e3 1e3]  NominalFrequency=60  UnbalancedPower=off  ActivePower=2200000  InductivePower=660e6  CapacitivePower=0  Pabc=[10e3 9e3 11e3]  QLabc=[100 90 110]  QCabc=[100 90 110]  Pabcp=[10e3 9e3 11e3]  QLabcp=[100 90 110]  QCabcp=[100 90 110]  Measurements=None  LoadType=constant Z
  LG3-LMO 104km : spsDistributedParametersLineLib/Distributed Parameters Line  Phases=3  Length=104  Frequency=60  Resistance="[0.01273  0.3864]"  Inductance="[0.9337e-3  4.1264e-3]"  Capacitance=[12.74e-9 7.751e-9]  x1=[-0.0006 -1.05438822074552e-09 0 0;-0.000525 -1.08953243572202e-09 0 0;-0.00045 -1.1238056951398e-09 0 0;-0.000375 -1.1571806014797e-09 517925.153195555 -372929.642144719;-0.0003 -1.18963047535223e-09 528261.054070984 -358138.485674645;-0.000225 -1.22112937682472e-09 538174.671142455 -343061.038778826;-0.00015 -1.25165212615728e-09 547658.079616163 -327709.354137617;-7.5e-05 -1.28117432393111e-09 556703.698600475 -312095.703652832]  x2=[-0.0006 6.01002737875507e-09 0 0;-0.000525 5.91501739323267e-09 0 0;-0.00045 5.81527903330891e-09 0 0;-0.000375 5.71089202830268e-09 463443.996877882 -442193.458727664;-0.0003 5.60193982358861e-09 475759.806920961 -428914.853919962;-0.000225 5.48850951389211e-09 487695.301853757 -415293.381140653;-0.00015 5.37069177366722e-09 499240.940624239 -401339.929186663;-7.5e-05 5.24858078461279e-09 510387.493825429 -387065.652233987]  x3=[-0.0006 1.99618173674951e-11 0 0;-0.000525 2.09800609958677e-11 0 0;-0.00045 2.19815334844858e-11 0 0;-0.000375 2.29654342715652e-11 -131.246118914113 -82.6228309095284;-0.0003 2.39309768418708e-11 -128.857332347106 -86.299842811043;-0.000225 2.48773893554452e-11 -126.365539200204 -89.9078679386463;-0.00015 2.58039152646057e-11 -123.772731374723 -93.444022092256;-7.5e-05 2.67098139187169e-11 -121.080981521567 -96.9054785243466]  x4=[-0.0006 -1.42656645126995e-11 0 0;-0.000525 -1.53794675845548e-11 0 0;-0.00045 -1.64809765453367e-11 0 0;-0.000375 -1.75693108656356e-11 3539.61351587993 -3162.16565183061;-0.0003 -1.86436005476481e-11 3627.59428501917 -3060.83488284544;-0.000225 -1.97029868206394e-11 3712.67521079103 -2957.05732928726;-0.00015 -2.07466228274321e-11 3794.78828080521 -2850.91594934455;-7.5e-05 -2.17736743013705e-11 3873.86785512993 -2742.4955908124]  x5=0.000588163229675572  V1=ones(3,3)  V2=ones(3,3)  I1=ones(3,3)  I2=ones(3,3)  nHarmo=1  Measurements=None  Decoupling=off  VsMag0=[ 1 1 1]  VrMag0=[ 1 1 1]  VsAngle0=[0 -120 120]  VrAngle0=[0 -120 120]  IsMag0=[ 1 1 1]  IrMag0=[ 1 1 1]  IsAngle0=[0 -120 120]  IrAngle0=[0 -120 120]
      settings: AttributesFormatString=\n  LibrarySourceBlock=sps_lib/Power Grid Elements/Distributed Parameters Line
  LG31-200 MVA : spsSynchronousMachinepuStandardLib/Synchronous Machine pu Standard  PresetModel=No  MechanicalLoad=Mechanical power Pm  ShowDetailedParameters=on  RotorType=Salient-pole  Units=per unit standard parameters  MeasurementBus=off  NominalParameters="[200E6  13800   60 ]"  Reactances1=[ 31 32 33 34 35 36 37 ]  Reactances2=[ 1.305, 0.296, 0.252, 0.474, 0.243, 0.18 ]  dAxisTimeConstants=Short-circuit  qAxisTimeConstants=Open-circuit  TimeConstants1=[]  TimeConstants2=[]  TimeConstants3=[]  TimeConstants4=[]  TimeConstants5=[ 1.01, 0.053, 0.1 ]  TimeConstants6=[]  TimeConstants7=[]  TimeConstants8=[]  StatorResistance=2.8544e-3  Mechanical="[ 3.2  0  32]"  PolePairs=32  InitialConditions=[0 -67.6291 0.902477 0.902477 0.902477 -4.2812 -124.281 115.719 1.45511]  SetSaturation=off  Saturation=[0.6404,0.7127,0.8441,0.9214,0.9956,1.082,1.19,1.316,1.457;0.7,0.7698,0.8872,0.9466,0.9969,1.046,1.1,1.151,1.201]  LoadFlowParameters=[1 180000000 0 0 0]  TsPowergui=0  TsBlock=-1  IterativeModel=Trapezoidal non iterative  IterativeDiscreteModel=Trapezoidal non iterative  BusType=PV  Pref=180000000  Qref=0  Qmin=-Inf  Qmax=Inf  PLF=0  QLF=0
  LG3_2200 MVA : spsSynchronousMachinepuStandardLib/Synchronous Machine pu Standard  PresetModel=No  MechanicalLoad=Mechanical power Pm  ShowDetailedParameters=on  RotorType=Salient-pole  Units=per unit standard parameters  MeasurementBus=off  NominalParameters="[2200E6  13800   60 ]"  Reactances1=[ 31 32 33 34 35 36 37 ]  Reactances2=[ 1.305, 0.296, 0.252, 0.474, 0.243, 0.18 ]  dAxisTimeConstants=Short-circuit  qAxisTimeConstants=Open-circuit  TimeConstants1=[]  TimeConstants2=[]  TimeConstants3=[]  TimeConstants4=[]  TimeConstants5=[ 1.01, 0.053, 0.1 ]  TimeConstants6=[]  TimeConstants7=[]  TimeConstants8=[]  StatorResistance=2.8544e-3  Mechanical="[ 3.2  0  32]"  PolePairs=32  InitialConditions=[0 -70.0065 0.820496 0.820496 0.820496 -4.90643 -124.906 115.094 1.38903]  SetSaturation=off  Saturation=[0.6404,0.7127,0.8441,0.9214,0.9956,1.082,1.19,1.316,1.457;0.7,0.7698,0.8872,0.9466,0.9969,1.046,1.1,1.151,1.201]  LoadFlowParameters=[1 1800000000 0 0 0]  TsPowergui=0  TsBlock=-1  IterativeModel=Trapezoidal non iterative  IterativeDiscreteModel=Trapezoidal non iterative  BusType=PV  Pref=1800000000  Qref=0  Qmin=-Inf  Qmax=Inf  PLF=0  QLF=0
  LG4 660 Mvar : spsThreePhaseSeriesRLCLoadLib/Three-Phase Series RLC Load  LConnTagsString=A|B|C  Configuration=Y (grounded)  NominalVoltage=735e3  Vabc=[1e3 1e3 1e3]  Vabcp=[1e3 1e3 1e3]  NominalFrequency=60  UnbalancedPower=off  ActivePower=2200000  InductivePower=660e6  CapacitivePower=0  Pabc=[10e3 9e3 11e3]  QLabc=[100 90 110]  QCabc=[100 90 110]  Pabcp=[10e3 9e3 11e3]  QLabcp=[100 90 110]  QCabcp=[100 90 110]  Measurements=None  LoadType=constant Z
  LG4-2700 MVA : spsSynchronousMachinepuStandardLib/Synchronous Machine pu Standard  PresetModel=No  MechanicalLoad=Mechanical power Pm  ShowDetailedParameters=on  RotorType=Salient-pole  Units=per unit standard parameters  MeasurementBus=off  NominalParameters="[2700E6  13800   60 ]"  Reactances1=[ 31 32 33 34 35 36 37 ]  Reactances2=[ 1.305, 0.296, 0.252, 0.474, 0.243, 0.18 ]  dAxisTimeConstants=Short-circuit  qAxisTimeConstants=Open-circuit  TimeConstants1=[]  TimeConstants2=[]  TimeConstants3=[]  TimeConstants4=[]  TimeConstants5=[ 1.01, 0.053, 0.1 ]  TimeConstants6=[]  TimeConstants7=[]  TimeConstants8=[]  StatorResistance=2.8544e-3  Mechanical="[ 3.7  0  32]"  PolePairs=32  InitialConditions=[0 -69.506 0.926038 0.926038 0.926038 -2.40174 -122.402 117.598 1.38766]  SetSaturation=off  Saturation=[0.6404,0.7127,0.8441,0.9214,0.9956,1.082,1.19,1.316,1.457;0.7,0.7698,0.8872,0.9466,0.9969,1.046,1.1,1.151,1.201]  LoadFlowParameters=[1 2500000000 0 0 0]  TsPowergui=0  TsBlock=-1  IterativeModel=Trapezoidal non iterative  IterativeDiscreteModel=Trapezoidal non iterative  BusType=PV  Pref=2500000000  Qref=0  Qmin=-Inf  Qmax=Inf  PLF=0  QLF=0
  LG4-LMO 3*118km : spsDistributedParametersLineLib/Distributed Parameters Line  Phases=3  Length=118  Frequency=60  Resistance="[0.01273  0.3864]/3"  Inductance="[0.9337e-3  4.1264e-3]/3"  Capacitance=[12.74e-9 7.751e-9]*3  x1=[-0.000675 -9.28207303145838e-10 442233.573338341 -460179.103702576;-0.0006 -9.80570386446272e-10 455066.323387897 -447492.94954335;-0.000525 -1.03214961678301e-09 467535.300381286 -434449.07636713;-0.00045 -1.08290376250851e-09 479630.536809079 -421057.911246556;-0.000375 -1.13279225153525e-09 491342.363924341 -407330.158874133;-0.0003 -1.18177520376841e-09 502661.419471672 -393276.793005067;-0.000225 -1.22981346298544e-09 513578.655171255 -378909.047685009;-0.00015 -1.27686862813694e-09 524085.34395191 -364238.408269735;-7.5e-05 -1.32290308404386e-09 534173.086927386 -349276.602243925]  x2=[-0.000675 6.1002330403474e-09 410578.900355497 -491671.191825551;-0.0006 6.01002737875507e-09 424314.599421719 -479867.339288603;-0.000525 5.91501739323267e-09 437711.107889395 -467679.888142844;-0.00045 5.81527903330891e-09 450757.716794629 -455118.580850246;-0.000375 5.71089202830268e-09 463443.996877882 -442193.458727664;-0.0003 5.60193982358861e-09 475759.806920961 -428914.853919962;-0.000225 5.48850951389211e-09 487695.301853757 -415293.381140653;-0.00015 5.37069177366722e-09 499240.940624239 -401339.929186663;-7.5e-05 5.24858078461279e-09 510387.493825429 -387065.652233987]  x3=[-0.000675 4.29466804975082e-11 2132.87241011305 -3249.81810531096;-0.0006 4.55628319667384e-11 2223.89341215585 -3188.22149349401;-0.000525 4.81425612052291e-11 2313.13666783167 -3124.0762661966;-0.00045 5.06838060168982e-11 2400.53083744741 -3057.43370013195;-0.000375 5.31845349695256e-11 2486.00605944105 -2988.34706834772;-0.0003 5.56427490186491e-11 2569.49400622794 -2916.8715976403;-0.000225 5.80564831055697e-11 2650.92793882083 -2843.06442440736;-0.00015 6.04238077281897e-11 2730.24276017998 -2766.98454897389;-7.5e-05 6.27428304834269e-11 2807.37506725076 -2688.69278842826]  x4=[-0.000675 -2.30327144035067e-11 6469.81651370838 -7978.71819622874;-0.0006 -2.60640182100971e-11 6692.79371784135 -7792.62324242263;-0.000525 -2.90744868393232e-11 6910.42080507946 -7600.29898482766;-0.00045 -3.20617137686245e-11 7122.52380765897 -7401.89916451269;-0.000375 -3.50233110544998e-11 7328.93317368491 -7197.58237925847;-0.0003 -3.79569112413928e-11 7529.48390266824 -6987.51195677697;-0.000225 -4.08601692541997e-11 7724.01567742474 -6771.85582414974;-0.00015 -4.37307642728863e-11 7912.37299223012 -6550.78637358956;-7.5e-05 -4.65664015877162e-11 8094.40527712887 -6324.48032463272]  x5=0.000667339049054976  V1=ones(3,3)  V2=ones(3,3)  I1=ones(3,3)  I2=ones(3,3)  nHarmo=1  Measurements=None  Decoupling=off  VsMag0=[ 1 1 1]  VrMag0=[ 1 1 1]  VsAngle0=[0 -120 120]  VrAngle0=[0 -120 120]  IsMag0=[ 1 1 1]  IrMag0=[ 1 1 1]  IsAngle0=[0 -120 120]  IrAngle0=[0 -120 120]
      settings: AttributesFormatString=\n  LibrarySourceBlock=sps_lib/Power Grid Elements/Distributed Parameters Line
  LMO 330 Mvar : spsThreePhaseSeriesRLCLoadLib/Three-Phase Series RLC Load  LConnTagsString=A|B|C  Configuration=Y (grounded)  NominalVoltage=735e3  Vabc=[1e3 1e3 1e3]  Vabcp=[1e3 1e3 1e3]  NominalFrequency=60  UnbalancedPower=off  ActivePower=1100000  InductivePower=330e6  CapacitivePower=0  Pabc=[10e3 9e3 11e3]  QLabc=[100 90 110]  QCabc=[100 90 110]  Pabcp=[10e3 9e3 11e3]  QLabcp=[100 90 110]  QCabcp=[100 90 110]  Measurements=None  LoadType=constant Z
  LMO-ALB 3*218km : spsDistributedParametersLineLib/Distributed Parameters Line  Phases=3  Length=218  Frequency=60  Resistance="[0.01273  0.3864]/3"  Inductance="[0.9337e-3  4.1264e-3]/3"  Capacitance=[12.74e-9 7.751e-9]*3  x1=[-0.001275 6.64110127154542e-09 0 0;-0.0012 6.59159221317464e-09 0 0;-0.001125 6.5368139368434e-09 0 0;-0.00105 6.47681023146765e-09 0 0;-0.000975 6.41162906309139e-09 0 0;-0.0009 6.3413225365433e-09 0 0;-0.000825 6.26594685378499e-09 382134.113224537 -514090.671982271;-0.00075 6.18556226898397e-09 396514.990798398 -503082.009934575;-0.000675 6.1002330403474e-09 410578.900355497 -491671.191825551;-0.0006 6.01002737875507e-09 424314.599421719 -479867.339288603;-0.000525 5.91501739323267e-09 437711.107889395 -467679.888142844;-0.00045 5.81527903330891e-09 450757.716794629 -455118.580850246;-0.000375 5.71089202830268e-09 463443.996877882 -442193.458727664;-0.0003 5.60193982358861e-09 475759.806920961 -428914.853919962;-0.000225 5.48850951389211e-09 487695.301853757 -415293.381140653;-0.00015 5.37069177366722e-09 499240.940624239 -401339.929186663;-7.5e-05 5.24858078461279e-09 510387.493825429 -387065.652233987]  x2=[-0.001275 2.18331184649544e-08 0 0;-0.0012 2.17333244107843e-08 0 0;-0.001125 2.16161570696113e-08 0 0;-0.00105 2.14817101032151e-08 0 0;-0.000975 2.13300909864435e-08 0 0;-0.0009 2.11614209212988e-08 0 0;-0.000825 2.09758347400501e-08 256872.501303858 -581628.877216981;-0.00075 2.07734807974513e-08 273212.791420058 -574134.44189225;-0.000675 2.0554520852148e-08 289334.679411093 -566181.052279222;-0.0006 2.03191299373701e-08 305225.277686376 -557775.066195863;-0.000525 2.00674962210134e-08 320871.883544779 -548923.203258832;-0.00045 1.97998208552206e-08 336261.989328982 -539632.539511922;-0.000375 1.95163178155836e-08 351383.292423895 -529910.501769581;-0.0003 1.92172137300945e-08 366223.70509119 -519764.861680028;-0.000225 1.89027476979828e-08 380771.364132046 -509203.729512717;-0.00015 1.8573171098583e-08 395014.640370411 -498235.547675111;-7.5e-05 1.82287473903861e-08 408942.147949191 -486869.083963954]  x3=[-0.001275 6.87788516620885e-11 0 0;-0.0012 7.2180760026208e-11 0 0;-0.001125 7.55249681951653e-11 0 0;-0.00105 7.88088028601181e-11 0 0;-0.000975 8.20296389738797e-11 0 0;-0.0009 8.51849018493411e-11 0 0;-0.000825 8.82720692176368e-11 558.937753073732 -1417.04584856669;-0.00075 9.12886732444079e-11 598.774931612781 -1400.67750101596;-0.000675 9.4232302502551e-11 638.133458633062 -1383.189473302;-0.0006 9.71006038998761e-11 676.981871530282 -1364.5957450866;-0.000525 9.98912845601328e-11 715.28911547757 -1344.91117991159;-0.00045 1.026021136559e-10 753.024568250236 -1324.15151331718;-0.000375 1.05230924191875e-10 790.158064704704 -1302.33334026323;-0.0003 1.07775614737139e-10 826.659920892072 -1279.47410186345;-0.000225 1.10234151105004e-10 862.500957787 -1255.59207144324;-0.00015 1.12604567979115e-10 897.652524612979 -1230.70633993232;-7.5e-05 1.14884970484491e-10 932.086521745328 -1204.8368006037]  x4=[-0.001275 4.24638038752998e-11 0 0;-0.0012 3.91998566112015e-11 0 0;-0.001125 3.59045735815061e-11 0 0;-0.00105 3.2580588985048e-11 0 0;-0.000975 2.92305599642551e-11 0 0;-0.0009 2.58571644810692e-11 0 0;-0.000825 2.24630991762251e-11 4744.07291566573 -11636.8846137311;-0.00075 1.90510772135965e-11 5071.15764281629 -11498.115607074;-0.000675 1.56238261113346e-11 5394.18856413849 -11350.1551827277;-0.0006 1.21840855615318e-11 5712.90745365637 -11193.1216179914;-0.000525 8.73460524015387e-12 6027.05953236621 -11027.1404430943;-0.00045 5.27814260899092e-12 6336.39367190298 -10852.3443408479;-0.000375 1.81746071138465e-12 6640.66259528851 -10668.8730405818;-0.0003 -1.64467403650624e-12 6939.62307460091 -10476.8732064463;-0.000225 -5.10549405713669e-12 7233.03612540726 -10276.4983201712;-0.00015 -8.56223282393455e-12 7520.66719780413 -10067.9085583745;-7.5e-05 -1.20121270728195e-11 7802.28636391314 -9851.27066452052]  x5=0.00123288061605072  V1=ones(3,3)  V2=ones(3,3)  I1=ones(3,3)  I2=ones(3,3)  nHarmo=1  Measurements=None  Decoupling=off  VsMag0=[ 1 1 1]  VrMag0=[ 1 1 1]  VsAngle0=[0 -120 120]  VrAngle0=[0 -120 120]  IsMag0=[ 1 1 1]  IrMag0=[ 1 1 1]  IsAngle0=[0 -120 120]  IrAngle0=[0 -120 120]
      settings: AttributesFormatString=\n  LibrarySourceBlock=sps_lib/Power Grid Elements/Distributed Parameters Line
  LMO7 : spsThreePhaseVIMeasurementLib/Three-Phase V-I Measurement  VoltageMeasurement=no  SetLabelV=on  LabelV=Vabc_LMO7  Vpu=on  VpuLL=off  CurrentMeasurement=no  SetLabelI=off  LabelI=A1  Ipu=off  Pbase=100e6  Vbase=735e3  OutputType=Magnitude  PhasorSimulation=off  PSBequivalent=0
  LVD 990 Mvar : spsThreePhaseSeriesRLCLoadLib/Three-Phase Series RLC Load  LConnTagsString=A|B|C  Configuration=Y (grounded)  NominalVoltage=735e3  Vabc=[1e3 1e3 1e3]  Vabcp=[1e3 1e3 1e3]  NominalFrequency=60  UnbalancedPower=off  ActivePower=3300000  InductivePower=990e6  CapacitivePower=0  Pabc=[10e3 9e3 11e3]  QLabc=[100 90 110]  QCabc=[100 90 110]  Pabcp=[10e3 9e3 11e3]  QLabcp=[100 90 110]  QCabcp=[100 90 110]  Measurements=None  LoadType=constant Z
  LVD-MTL 3*260km : spsDistributedParametersLineLib/Distributed Parameters Line  Phases=3  Length=260  Frequency=60  Resistance="[0.01273  0.3864]/3"  Inductance="[0.9337e-3  4.1264e-3]/3"  Capacitance=[12.74e-9 7.751e-9]*3  x1=[-0.0015 7.52904676811522e-08 -60766.0885085607 -643710.8080293;-0.001425 7.5149442529736e-08 -42543.7444110895 -645171.399881521;-0.00135 7.49483440637865e-08 -24287.3914952771 -646116.25158813;-0.001275 7.46873330383405e-08 -6011.62361031296 -646544.60784913;-0.0012 7.43666181016182e-08 12268.9498745843 -646456.126243079;-0.001125 7.39864556282329e-08 30539.7157486731 -645850.87750082;-0.00105 7.35471495142491e-08 48786.0686412657 -644729.345448937;-0.000975 7.30490509342527e-08 66993.4226970384 -643092.426622991;-0.0009 7.24925580606275e-08 85147.2232357407 -640941.429550848;-0.000825 7.18781157452619e-08 103232.958386985 -638278.073706654;-0.00075 7.12062151639416e-08 121236.170690811 -635104.488136321;-0.000675 7.04773934237109e-08 139142.468654763 -631423.209755596;-0.0006 6.96922331335175e-08 156937.538258224 -627237.181322092;-0.000525 6.88513619384841e-08 174607.154394826 -622549.74908289;-0.00045 6.79554520181783e-08 192137.192243783 -617364.660099601;-0.000375 6.70052195492824e-08 209513.638561059 -611686.059253025;-0.0003 6.60014241330931e-08 226722.602881335 -605518.485929792;-0.000225 6.49448681883074e-08 243750.328621839 -598866.870393651;-0.00015 6.38363963095818e-08 260583.204079149 -591736.529844287;-7.5e-05 6.2676894592376e-08 277207.773310174 -584133.164166838]  x2=[-0.0015 1.11983560483815e-07 -284434.156182368 -570661.101567477;-0.001425 1.11648980639992e-07 -268187.556421174 -578474.126624328;-0.00135 1.11225150309332e-07 -251726.571630784 -585824.728315307;-0.001275 1.10712408295317e-07 -235064.360470578 -592707.03068189;-0.0012 1.10111164476067e-07 -218214.242457218 -599115.532116867;-0.001125 1.09421899476692e-07 -201189.687317227 -605045.109762245;-0.00105 1.08645164285087e-07 -184004.3042195 -610491.02360438;-0.000975 1.07781579811479e-07 -166671.83089634 -615448.920263071;-0.0009 1.06831836392083e-07 -149206.122661726 -619914.836471588;-0.000825 1.05796693237257e-07 -131621.141335587 -623885.202244845;-0.00075 1.04676977824601e-07 -113930.944082935 -627356.84373319;-0.000675 1.03473585237484e-07 -96149.6721767847 -630326.985759538;-0.0006 1.02187477449527e-07 -78291.5396938359 -632793.254037795;-0.000525 1.00819682555617e-07 -60370.8221519566 -634753.677070836;-0.00045 9.93712939500652e-08 -42401.8450985535 -636206.687726483;-0.000375 9.78434694525616e-08 -24398.9726589487 -637151.124490251;-0.0003 9.62374303826328e-08 -6376.59605391708 -637586.23239384;-0.000225 9.45544605833383e-08 11650.8779044348 -637511.663618651;-0.00015 9.27959053949852e-08 29669.0383292544 -636927.47777382;-7.5e-05 9.09631705796843e-08 47663.481778785 -635834.141848573]  x3=[-0.0015 3.86105231526987e-10 283.845435906203 550.505795113289;-0.001425 3.94651876670943e-10 268.169144866339 558.310803130396;-0.00135 4.02883043143064e-10 252.278483515195 565.669506033924;-0.001275 4.10792151074814e-10 236.186154604318 572.576021389361;-0.0012 4.18372878046326e-10 219.905022095221 579.024828234007;-0.001125 4.25619164140446e-10 203.448100876119 585.01077149034;-0.00105 4.32525216786945e-10 186.828546358038 590.529066086908;-0.000975 4.39085515393002e-10 170.059643958571 595.575300783443;-0.0009 4.45294815756287e-10 153.154798481724 600.145441697141;-0.000825 4.51148154257096e-10 136.127523402317 604.235835527278;-0.00075 4.5664085182619e-10 118.991430063523 607.843212475614;-0.000675 4.61768517685174e-10 101.760216796166 610.96468886021;-0.0006 4.66527052856415e-10 84.4476579684858 613.597769420603;-0.000525 4.70912653439706e-10 67.0675929751182 615.740349312483;-0.00045 4.74921813653043e-10 49.6339151740949 617.390715790266;-0.000375 4.78551328635093e-10 32.1605607807058 618.54754957624;-0.0003 4.81798297007112e-10 14.6614977271016 619.209925915179;-0.000225 4.84660123192266e-10 -2.8492855034571 619.37731531357;-0.00015 4.87134519490488e-10 -20.3577910587799 619.04958396289;-7.5e-05 4.89219507907237e-10 -37.850022907415 618.226993846567]  x4=[-0.0015 3.23358890257174e-10 -6356.55576531234 -13234.8737869072;-0.001425 3.18634308620088e-10 -5979.85814727471 -13409.2877766837;-0.00135 3.13655015591959e-10 -5598.38032212904 -13572.9825869805;-0.001275 3.08424991543449e-10 -5212.42723741195 -13725.8273626709;-0.0012 3.0294841727576e-10 -4822.30741811409 -13867.6999219798;-0.001125 2.97229670678566e-10 -4428.33272004996 -13998.486854154;-0.00105 2.91273323230399e-10 -4030.81808056519 -14118.083610121;-0.000975 2.85084136344273e-10 -3630.0812667804 -14226.3945860639;-0.0009 2.78667057561486e-10 -3226.44262157305 -14323.333199846;-0.000825 2.72027216596634e-10 -2820.22480750024 -14408.8219602224;-0.00075 2.65169921236991e-10 -2411.75254886721 -14482.7925287861;-0.000675 2.58100653099546e-10 -2001.35237214766 -14545.1857745966;-0.0006 2.50825063249087e-10 -1589.35234496353 -14595.9518214476;-0.000525 2.43348967680818e-10 -1176.08181383275 -14635.0500877381;-0.00045 2.35678342671149e-10 -761.871140894645 -14662.4493189122;-0.000375 2.27819320000348e-10 -347.051439823528 -14678.1276124438;-0.0003 2.19778182050891e-10 68.0456888585197 -14682.0724353449;-0.000225 2.11561356785422e-10 483.088422858027 -14674.2806341844;-0.00015 2.03175412608336e-10 897.744983363803 -14654.758437609;-7.5e-05 1.94627053115099e-10 1311.68390026584 -14623.5214513639]  x5=0.00147040807418893  V1=ones(3,3)  V2=ones(3,3)  I1=ones(3,3)  I2=ones(3,3)  nHarmo=1  Measurements=None  Decoupling=off  VsMag0=[ 1 1 1]  VrMag0=[ 1 1 1]  VsAngle0=[0 -120 120]  VrAngle0=[0 -120 120]  IsMag0=[ 1 1 1]  IrMag0=[ 1 1 1]  IsAngle0=[0 -120 120]  IrAngle0=[0 -120 120]
      settings: AttributesFormatString=\n  LibrarySourceBlock=sps_lib/Power Grid Elements/Distributed Parameters Line
  LVD7 : spsThreePhaseVIMeasurementLib/Three-Phase V-I Measurement  VoltageMeasurement=no  SetLabelV=on  LabelV=Vabc_LVD7  Vpu=on  VpuLL=off  CurrentMeasurement=no  SetLabelI=off  LabelI=A1  Ipu=off  Pbase=100e6  Vbase=735e3  OutputType=Magnitude  PhasorSimulation=off  PSBequivalent=0
  Load Flow Bus1 : spsLoadFlowBusLib/Load Flow Bus  LConnTagsString=a  Phases=single  Connectors=on one side  ID=LG31_13.8  Vbase=13.8e3  Vref=1  Vangle=0  VLF=1  VLFb=1  VLFc=1  angleLF=-0.0351  angleLFb=0  angleLFc=0
      settings: AttributesFormatString=%<ID>\n%<Vbase>V\n%<VLF>pu\n%<angleLF>deg.
  Load Flow Bus10 : spsLoadFlowBusLib/Load Flow Bus  LConnTagsString=a  Phases=single  Connectors=on one side  ID=LVD7  Vbase=735e3  Vref=1  Vangle=0  VLF=1.05  VLFb=1  VLFc=1  angleLF=-12.02  angleLFb=0  angleLFc=0
      settings: AttributesFormatString=%<ID>\n%<Vbase>V\n%<VLF>pu\n%<angleLF>deg.
  Load Flow Bus11 : spsLoadFlowBusLib/Load Flow Bus  LConnTagsString=a  Phases=single  Connectors=on one side  ID=CHM7  Vbase=735e3  Vref=1  Vangle=0  VLF=1.047  VLFb=1  VLFc=1  angleLF=-4.064  angleLFb=0  angleLFc=0
      settings: AttributesFormatString=%<ID>\n%<Vbase>V\n%<VLF>pu\n%<angleLF>deg.
  Load Flow Bus12 : spsLoadFlowBusLib/Load Flow Bus  LConnTagsString=a  Phases=single  Connectors=on one side  ID=LG47  Vbase=735e3  Vref=1  Vangle=0  VLF=1.004  VLFb=1  VLFc=1  angleLF=20.71  angleLFb=0  angleLFc=0
      settings: AttributesFormatString=%<ID>\n%<Vbase>V\n%<VLF>pu\n%<angleLF>deg.
  Load Flow Bus2 : spsLoadFlowBusLib/Load Flow Bus  LConnTagsString=a  Phases=single  Connectors=on one side  ID=LG3_13.8  Vbase=13.8e3  Vref=1  Vangle=0  VLF=1  VLFb=1  VLFc=1  angleLF=-0.6025  angleLFb=0  angleLFc=0
      settings: AttributesFormatString=%<ID>\n%<Vbase>V\n%<VLF>pu\n%<angleLF>deg.
  Load Flow Bus3 : spsLoadFlowBusLib/Load Flow Bus  LConnTagsString=a  Phases=single  Connectors=on one side  ID=LG4_13.8  Vbase=13.8e3  Vref=1  Vangle=0  VLF=1  VLFb=1  VLFc=1  angleLF=-3.293  angleLFb=0  angleLFc=0
      settings: AttributesFormatString=%<ID>\n%<Vbase>V\n%<VLF>pu\n%<angleLF>deg.
  Load Flow Bus4 : spsLoadFlowBusLib/Load Flow Bus  LConnTagsString=a  Phases=single  Connectors=on one side  ID=LG2_13.8  Vbase=13.8e3  Vref=1  Vangle=0  VLF=1  VLFb=1  VLFc=1  angleLF=0  angleLFb=0  angleLFc=0
      settings: AttributesFormatString=%<ID>\n%<Vbase>V\n%<VLF>pu\n%<angleLF>deg.
  Load Flow Bus5 : spsLoadFlowBusLib/Load Flow Bus  LConnTagsString=a  Phases=single  Connectors=on one side  ID=LG27  Vbase=735e3  Vref=1  Vangle=0  VLF=1  VLFb=1  VLFc=1  angleLF=23.57  angleLFb=0  angleLFc=0
      settings: AttributesFormatString=%<ID>\n%<Vbase>V\n%<VLF>pu\n%<angleLF>deg.
  Load Flow Bus6 : spsLoadFlowBusLib/Load Flow Bus  LConnTagsString=a  Phases=single  Connectors=on one side  ID=LG37  Vbase=735e3  Vref=1  Vangle=0  VLF=0.994  VLFb=1  VLFc=1  angleLF=24.1  angleLFb=0  angleLFc=0
      settings: AttributesFormatString=%<ID>\n%<Vbase>V\n%<VLF>pu\n%<angleLF>deg.
  Load Flow Bus7 : spsLoadFlowBusLib/Load Flow Bus  LConnTagsString=a  Phases=single  Connectors=on one side  ID=LMO7  Vbase=735e3  Vref=1  Vangle=0  VLF=1.016  VLFb=1  VLFc=1  angleLF=17.31  angleLFb=0  angleLFc=0
      settings: AttributesFormatString=%<ID>\n%<Vbase>V\n%<VLF>pu\n%<angleLF>deg.
  Load Flow Bus8 : spsLoadFlowBusLib/Load Flow Bus  LConnTagsString=a  Phases=single  Connectors=on one side  ID=NEM_ALB7  Vbase=735e3  Vref=1  Vangle=0  VLF=1.028  VLFb=1  VLFc=1  angleLF=8.928  angleLFb=0  angleLFc=0
      settings: AttributesFormatString=%<ID>\n%<Vbase>V\n%<VLF>pu\n%<angleLF>deg.
  Load Flow Bus9 : spsLoadFlowBusLib/Load Flow Bus  LConnTagsString=a  Phases=single  Connectors=on one side  ID=ABI_CHB7  Vbase=735e3  Vref=1  Vangle=0  VLF=1.046  VLFb=1  VLFc=1  angleLF=0.1334  angleLFb=0  angleLFc=0
      settings: AttributesFormatString=%<ID>\n%<Vbase>V\n%<VLF>pu\n%<angleLF>deg.
  NEM-ABI 6*236 : spsDistributedParametersLineLib/Distributed Parameters Line  Phases=3  Length=236  Frequency=60  Resistance="[0.01273  0.3864]/6"  Inductance="[0.9337e-3  4.1264e-3]/6"  Capacitance=[12.74e-9 7.751e-9]*6  x1=[-0.00135 2.1657809033025e-08 0 0;-0.001275 2.15818709673223e-08 0 0;-0.0012 2.14886806841821e-08 0 0;-0.001125 2.13783126784907e-08 0 0;-0.00105 2.12508551767434e-08 0 0;-0.000975 2.11064100665167e-08 0 0;-0.0009 2.09450928150217e-08 0 0;-0.000825 2.07670323768011e-08 284967.297433694 -571339.995920143;-0.00075 2.05723710906448e-08 301005.484998464 -563055.41594175;-0.000675 2.03612645658064e-08 316803.053384064 -554320.738078889;-0.0006 2.01338815576118e-08 332347.374256039 -545142.9446994;-0.000525 1.98904038325589e-08 347626.021722118 -535529.372390885;-0.00045 1.96310260230156e-08 362626.78226529 -525487.706095954;-0.000375 1.93559554716343e-08 377337.664507094 -515025.972969002;-0.0003 1.90654120656049e-08 391746.908793351 -504152.535959421;-0.000225 1.8759628060881e-08 405842.996594648 -492876.087126386;-0.00015 1.84388478965171e-08 419614.659714072 -481205.640690559;-7.5e-05 1.81033279992685e-08 433050.889294842 -469150.525828257]  x2=[-0.00135 3.84255814779631e-08 0 0;-0.001275 3.82701311151049e-08 0 0;-0.0012 3.8084088194986e-08 0 0;-0.001125 3.78676014374701e-08 0 0;-0.00105 3.76208438987588e-08 0 0;-0.000975 3.7344012833053e-08 0 0;-0.0009 3.70373295348711e-08 0 0;-0.000825 3.67010391621491e-08 124240.179514944 -633974.103134405;-0.00075 3.63354105402657e-08 142113.319168706 -630208.353511083;-0.000675 3.59407359471468e-08 159872.855609531 -625938.824972476;-0.0006 3.55173308796234e-08 177504.592135719 -621168.93051437;-0.000525 3.50655338012282e-08 194994.434206864 -615902.483117415;-0.00045 3.45857058716331e-08 212328.40071082 -610143.69269908;-0.000375 3.40782306579431e-08 229492.635139981 -603897.162748313;-0.0003 3.35435138280796e-08 246473.416667966 -597167.886645581;-0.000225 3.2981982826495e-08 263257.171117836 -589961.24367124;-0.00015 3.239408653248e-08 279830.481813085 -582282.994705418;-7.5e-05 3.17802949013372e-08 296180.100302722 -574139.277622856]  x3=[-0.00135 2.63717494457858e-10 0 0;-0.001275 2.71219120808335e-10 0 0;-0.0012 2.78503938743429e-10 0 0;-0.001125 2.85566124891145e-10 0 0;-0.00105 2.92400033847931e-10 0 0;-0.000975 2.99000202691529e-10 0 0;-0.0009 3.05361355347952e-10 0 0;-0.000825 3.11478406809096e-10 -663.961228467695 -1977.20263991295;-0.00075 3.17346467197616e-10 -607.798395729049 -1995.181663606;-0.000675 3.22960845675822e-10 -551.149698252484 -2011.56576960447;-0.0006 3.28317054195461e-10 -494.06042014001 -2026.34186070471;-0.000525 3.33410811085396e-10 -436.576197687054 -2039.49812512556;-0.00045 3.38238044474306e-10 -378.742982901506 -2051.02404595056;-0.000375 3.42794895545678e-10 -320.607006770389 -2060.91040953495;-0.0003 3.47077721622489e-10 -262.214742303512 -2069.14931287094;-0.000225 3.51083099079102e-10 -203.612867383657 -2075.73416990527;-0.00015 3.54807826078063e-10 -144.848227452997 -2080.65971680398;-7.5e-05 3.58248925129599e-10 -85.9677980655629 -2083.92201616023]  x4=[-0.00135 1.94568476592245e-10 0 0;-0.001275 1.88598203431706e-10 0 0;-0.0012 1.82477167752992e-10 0 0;-0.001125 1.76210262618371e-10 0 0;-0.00105 1.6980249769592e-10 0 0;-0.000975 1.63258995254877e-10 0 0;-0.0009 1.56584986070973e-10 0 0;-0.000825 1.49785805245034e-10 5549.38040349712 -25908.0748550784;-0.00075 1.42866887938183e-10 6279.59671941977 -25740.8357836483;-0.000675 1.3583376502705e-10 7004.79322180597 -25553.0198819408;-0.0006 1.28692058682481e-10 7724.39019966758 -25344.7772871139;-0.000525 1.21447477875256e-10 8437.81241819072 -25116.2744651118;-0.00045 1.14105813812426e-10 9144.48957856961 -24867.6940775942;-0.000375 1.06672935307912e-10 9843.85677389477 -24599.2348359195;-0.0003 9.91547840910628e-11 10535.3549407309 -24311.1113422978;-0.000225 9.15573700569308e-11 11218.4313060238 -24003.5539182416;-0.00015 8.388676646205e-11 11892.5398289784 -23676.8084204498;-7.5e-05 7.614910506957e-11 12557.1416375557 -23331.136044274]  x5=0.00133467809810995  V1=ones(3,3)  V2=ones(3,3)  I1=ones(3,3)  I2=ones(3,3)  nHarmo=1  Measurements=None  Decoupling=off  VsMag0=[ 1 1 1]  VrMag0=[ 1 1 1]  VsAngle0=[0 -120 120]  VrAngle0=[0 -120 120]  IsMag0=[ 1 1 1]  IrMag0=[ 1 1 1]  IsAngle0=[0 -120 120]  IrAngle0=[0 -120 120]
      settings: AttributesFormatString=\n  LibrarySourceBlock=sps_lib/Power Grid Elements/Distributed Parameters Line
  NEM-ALB 1980 Mvar : spsThreePhaseSeriesRLCLoadLib/Three-Phase Series RLC Load  LConnTagsString=A|B|C  Configuration=Y (grounded)  NominalVoltage=735e3  Vabc=[1e3 1e3 1e3]  Vabcp=[1e3 1e3 1e3]  NominalFrequency=60  UnbalancedPower=off  ActivePower=6600000  InductivePower=1980e6  CapacitivePower=0  Pabc=[10e3 9e3 11e3]  QLabc=[100 90 110]  QCabc=[100 90 110]  Pabcp=[10e3 9e3 11e3]  QLabcp=[100 90 110]  QCabcp=[100 90 110]  Measurements=None  LoadType=constant Z
  NEM-ALB7 : spsThreePhaseVIMeasurementLib/Three-Phase V-I Measurement  VoltageMeasurement=no  SetLabelV=on  LabelV=Vabc_NEM7  Vpu=on  VpuLL=off  CurrentMeasurement=no  SetLabelI=off  LabelI=A1  Ipu=off  Pbase=100e6  Vbase=735e3  OutputType=Magnitude  PhasorSimulation=off  PSBequivalent=0
  Regulators1 : Subsystem
  Regulators2 : Subsystem
  Regulators3 : Subsystem
  Regulators4 : Subsystem
  MTLa : PMIOPort  Side=Right
  MTLb : PMIOPort  Port=2  Side=Right
  MTLc : PMIOPort  Port=3  Side=Right
  CHM7a : PMIOPort  Port=4  Side=Right
  CHM7b : PMIOPort  Port=5  Side=Right
  CHM7c : PMIOPort  Port=6  Side=Right
  wires:
  Regulators2/1(Pm) -> LG3_2200 MVA/1
  Regulators4/2(Vf) -> LG4-2700 MVA/2
  Regulators4/1(Pm) -> LG4-2700 MVA/1
  Regulators3/2(Vf) -> LG31-200 MVA/2
  Regulators3/1(Pm) -> LG31-200 MVA/1
  Regulators2/2(Vf) -> LG3_2200 MVA/2
  LG3_2200 MVA/1 -> Regulators2/1(m)
  Regulators1/1(Pm) -> LG2_5500 MVA/1
  Regulators1/2(Vf) -> LG2_5500 MVA/2
  LG2_5500 MVA/1 -> Regulators1/1(m)
  LG31-200 MVA/1 -> Regulators3/1(m)
  LG4-2700 MVA/1 -> Regulators4/1(m)
  connections:
  LG2-NENI 3*279km/RConn1 -- "Cs NEM "/LConn1
  LG2-NENI 3*279km/RConn2 -- "Cs NEM "/LConn2
  LG2-NENI 3*279km/RConn3 -- "Cs NEM "/LConn3
  CHB-CHM 3*195km/RConn1 -- "Cs  CHMN "/LConn1
  CHB-CHM 3*195km/RConn2 -- "Cs  CHMN "/LConn2
  CHB-CHM 3*195km/RConn3 -- "Cs  CHMN "/LConn3
  Load Flow Bus2/LConn1 -- 2200 MVA 13.8 kV/735 kV/LConn1 -- LG3_2200 MVA/RConn1 -- 110 MW/LConn1
  2200 MVA 13.8 kV/735 kV/LConn2 -- LG3_2200 MVA/RConn2 -- 110 MW/LConn2
  2200 MVA 13.8 kV/735 kV/LConn3 -- LG3_2200 MVA/RConn3 -- 110 MW/LConn3
  Load Flow Bus1/LConn1 -- 200 MVA 13.8 kV/735 kV/LConn1 -- LG31-200 MVA/RConn1 -- 10 MW/LConn1
  200 MVA 13.8 kV/735 kV/LConn2 -- LG31-200 MVA/RConn2 -- 10 MW/LConn2
  200 MVA 13.8 kV/735 kV/LConn3 -- LG31-200 MVA/RConn3 -- 10 MW/LConn3
  Load Flow Bus6/LConn1 -- 2200 MVA 13.8 kV/735 kV/RConn1 -- 200 MVA 13.8 kV/735 kV/RConn1 -- LG3-LMO 104km/LConn1 -- LG3 660 Mvar/LConn1 -- LG2-LG3 155km/RConn1
  2200 MVA 13.8 kV/735 kV/RConn2 -- LG3 660 Mvar/LConn2 -- LG2-LG3 155km/RConn2 -- 200 MVA 13.8 kV/735 kV/RConn2 -- LG3-LMO 104km/LConn2
  LG3-LMO 104km/RConn1 -- LMO7/RConn1 -- LG4-LMO 3*118km/RConn1 -- LMO 330 Mvar/LConn1
  LG3-LMO 104km/RConn2 -- LMO7/RConn2 -- LG4-LMO 3*118km/RConn2 -- LMO 330 Mvar/LConn2
  LG3-LMO 104km/RConn3 -- LMO7/RConn3 -- LG4-LMO 3*118km/RConn3 -- LMO 330 Mvar/LConn3
  LG4-LMO 3*118km/LConn1 -- LG4 660 Mvar/LConn1 -- 2700 MVA 13.8 kV/735 kV/RConn1 -- Load Flow Bus12/LConn1
  LG4-LMO 3*118km/LConn2 -- 2700 MVA 13.8 kV/735 kV/RConn2 -- LG4 660 Mvar/LConn2
  LG4 660 Mvar/LConn3 -- 2700 MVA 13.8 kV/735 kV/RConn3 -- LG4-LMO 3*118km/LConn3
  Load Flow Bus3/LConn1 -- LG4-2700 MVA/RConn1 -- 2700 MVA 13.8 kV/735 kV/LConn1 -- 135 MW/LConn1
  LG4-2700 MVA/RConn2 -- 2700 MVA 13.8 kV/735 kV/LConn2 -- 135 MW/LConn2
  LG4-2700 MVA/RConn3 -- 2700 MVA 13.8 kV/735 kV/LConn3 -- 135 MW/LConn3
  Load Flow Bus4/LConn1 -- 5500 MVA 13.8 kV/735 kV/LConn1 -- LG2_5500 MVA/RConn1 -- 275 MW/LConn1
  5500 MVA 13.8 kV/735 kV/LConn2 -- LG2_5500 MVA/RConn2 -- 275 MW/LConn2
  LG2_5500 MVA/RConn3 -- 5500 MVA 13.8 kV/735 kV/LConn3 -- 275 MW/LConn3
  5500 MVA 13.8 kV/735 kV/RConn1 -- LG2-NENI 3*279km/LConn1 -- LG2-LG3 155km/LConn1 -- LG2 660 Mvar/LConn1 -- Load Flow Bus5/LConn1
  LG2-LG3 155km/LConn2 -- 5500 MVA 13.8 kV/735 kV/RConn2 -- LG2-NENI 3*279km/LConn2 -- LG2 660 Mvar/LConn2
  LG2-LG3 155km/LConn3 -- 5500 MVA 13.8 kV/735 kV/RConn3 -- LG2-NENI 3*279km/LConn3 -- LG2 660 Mvar/LConn3
  "Cs NEM "/RConn1 -- NEM-ALB7/LConn1 -- Cs ALB/RConn1
  "Cs NEM "/RConn2 -- NEM-ALB7/LConn2 -- Cs ALB/RConn2
  "Cs NEM "/RConn3 -- NEM-ALB7/LConn3 -- Cs ALB/RConn3
  LMO7/LConn1 -- LMO-ALB 3*218km/LConn1
  LMO7/LConn2 -- LMO-ALB 3*218km/LConn2
  Load Flow Bus7/LConn1 -- LMO7/LConn3 -- LMO-ALB 3*218km/LConn3
  Cs ALB/LConn1 -- LMO-ALB 3*218km/RConn1
  Cs ALB/LConn2 -- LMO-ALB 3*218km/RConn2
  Cs ALB/LConn3 -- LMO-ALB 3*218km/RConn3
  200 MVA 13.8 kV/735 kV/RConn3 -- LG3-LMO 104km/LConn3 -- LG3 660 Mvar/LConn3 -- LG2-LG3 155km/RConn3 -- 2200 MVA 13.8 kV/735 kV/RConn3
  Load Flow Bus8/LConn1 -- NEM-ABI 6*236/LConn1 -- NEM-ALB7/RConn1 -- NEM-ALB 1980 Mvar/LConn1
  NEM-ALB 1980 Mvar/LConn2 -- NEM-ALB7/RConn2 -- NEM-ABI 6*236/LConn2
  NEM-ALB 1980 Mvar/LConn3 -- NEM-ALB7/RConn3 -- NEM-ABI 6*236/LConn3
  NEM-ABI 6*236/RConn1 -- "Cs ABI+CHB "/LConn1
  NEM-ABI 6*236/RConn2 -- "Cs ABI+CHB "/LConn2
  NEM-ABI 6*236/RConn3 -- "Cs ABI+CHB "/LConn3
  "Cs ABI+CHB "/RConn1 -- ABI-CHB7/LConn1
  "Cs ABI+CHB "/RConn2 -- ABI-CHB7/LConn2
  "Cs ABI+CHB "/RConn3 -- ABI-CHB7/LConn3
  Load Flow Bus9/LConn1 -- ABI+CHB 1320 Mvar/LConn1 -- CHB-CHM 3*195km/LConn1 -- ABI-CHB 3*271km/LConn1 -- ABI-CHB7/RConn1
  ABI-CHB 3*271km/LConn2 -- ABI-CHB7/RConn2 -- ABI+CHB 1320 Mvar/LConn2 -- CHB-CHM 3*195km/LConn2
  ABI-CHB 3*271km/LConn3 -- ABI-CHB7/RConn3 -- ABI+CHB 1320 Mvar/LConn3 -- CHB-CHM 3*195km/LConn3
  ABI-CHB 3*271km/RConn1 -- "Cs LVDN "/LConn1
  ABI-CHB 3*271km/RConn2 -- "Cs LVDN "/LConn2
  ABI-CHB 3*271km/RConn3 -- "Cs LVDN "/LConn3
  "Cs LVDN "/RConn1 -- LVD7/LConn1
  "Cs LVDN "/RConn2 -- LVD7/LConn2
  "Cs LVDN "/RConn3 -- LVD7/LConn3
  "Cs LVDS "/LConn1 -- LVD 990 Mvar/LConn1 -- Load Flow Bus10/LConn1 -- LVD7/RConn1
  "Cs LVDS "/LConn2 -- LVD7/RConn2 -- LVD 990 Mvar/LConn2
  "Cs LVDS "/LConn3 -- LVD7/RConn3 -- LVD 990 Mvar/LConn3
  "Cs LVDS "/RConn1 -- LVD-MTL 3*260km/LConn1
  "Cs LVDS "/RConn2 -- LVD-MTL 3*260km/LConn2
  "Cs LVDS "/RConn3 -- LVD-MTL 3*260km/LConn3
  MTLa/RConn1 -- LVD-MTL 3*260km/RConn1
  MTLb/RConn1 -- LVD-MTL 3*260km/RConn2
  MTLc/RConn1 -- LVD-MTL 3*260km/RConn3
  "Cs  CHMN "/RConn1 -- CHM7/LConn1
  "Cs  CHMN "/RConn2 -- CHM7/LConn2
  "Cs  CHMN "/RConn3 -- CHM7/LConn3
  CHM 1320Mvar/LConn2 -- CHM7/RConn2 -- CHM7b/RConn1
  Load Flow Bus11/LConn1 -- CHM 1320Mvar/LConn3 -- CHM7c/RConn1 -- CHM7/RConn3
  CHM7a/RConn1 -- CHM 1320Mvar/LConn1 -- CHM7/RConn1
